simulink model "pidACC_bicycleModel"  (R2022a)
settings: Solver=FixedStepAuto  StartTime=0.0  StopTime=T  RelTol=1e-3
values from neighbouring files (symbols this model uses):
  o0_ego_1 = 0    [PreRun.m]
  o0_lead = 0    [PreRun.m]
  t_gap = 1.4    [PreRun.m]
  Ts = 1e-2    (= 0.01)    [PreRun.m]
  v0_ego_1 = 20/9    (= 2.22222222222)    [PreRun.m]
  v0_lead = 25/9    (= 2.77777777778)    [PreRun.m]
  x0_ego_1 = x0_lead - (10 + t_gap*v0_ego_1)    (= 56.8888888889)    [PreRun.m]
  x0_ego_2 = x0_ego_1 - (10 + t_gap*v0_ego_2)    (= 43.7777777778)    [PreRun.m]
  x0_lead = 70    [PreRun.m]
  y0_ego_1 = 0    [PreRun.m]
  y0_lead = 0    [PreRun.m]
undefined symbols (not defined in the file or in its folder): orient_kp
libraries: robotmobilelib x3
settings Model: Creator=The MathWorks, Inc.  LastModifiedBy=SAMEER TALWAR
settings SolverCC: AlgebraicLoopSolver=TrustRegion
settings DataIOCC: ReturnWorkspaceOutputs=off
settings DebuggingCC: UnconnectedInputMsg=warning  UnconnectedOutputMsg=warning  UnconnectedLineMsg=warning  SFMachineParentedDataDiag=warning  ArithmeticOperatorsInVariantConditions=warning
settings SFSimCC: SimUseLocalCustomCode=off  CustomCodeUndefinedFunction=UseInterfaceOnly
settings RTWCC: RTWUseLocalCustomCode=off
settings CodeAppCC: StateflowObjectComments=on

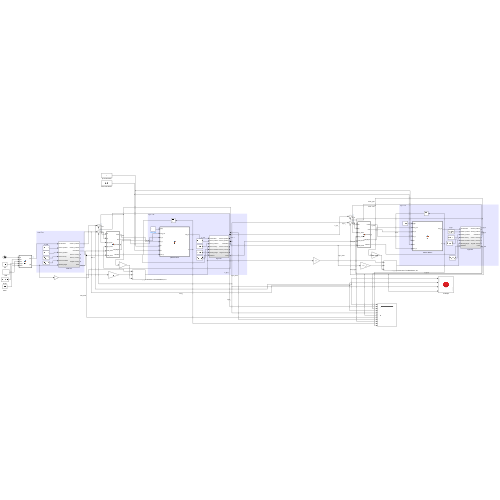
[thumbnail: Simulink's stored preview of the top-level diagram]
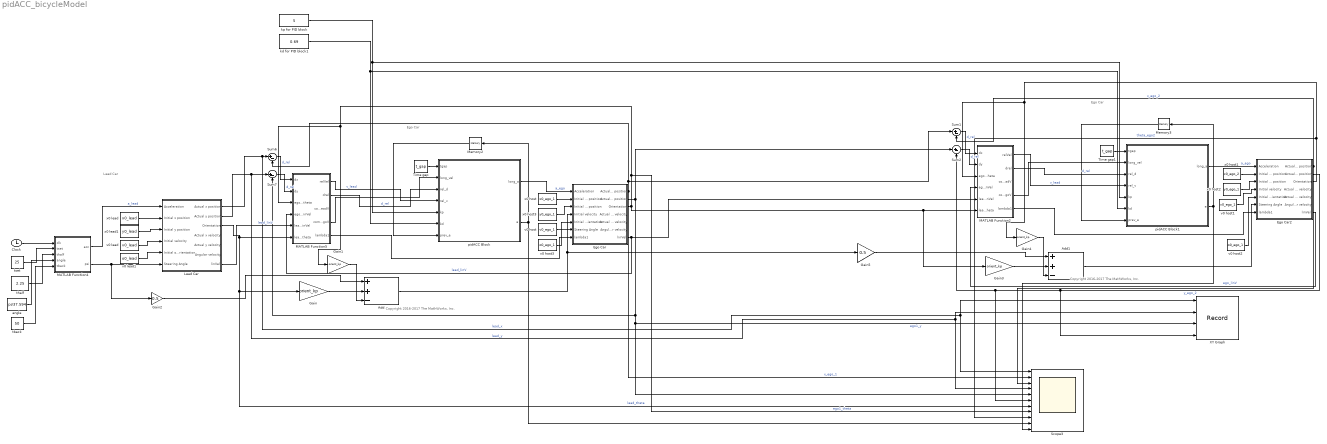
== system pidACC_bicycleModel ==
  note: Lead Car
  note: Ego Car
  note: Copyright 2016-2017 The MathWorks, Inc.
  note: Ego Car
  note: Copyright 2016-2017 The MathWorks, Inc.
  Add : Sum  Inputs=++-
  Add1 : Sum  Inputs=++-
  Clock : Clock
  Ego Car : Subsystem
  Ego Car2 : Subsystem
  Gain{,1,3..4} (4 alike) : Gain  Gain=orient_kp
  Gain2 : Gain  Gain=0.5
  Gain5 : Gain  Gain=0.5
  Lead Car : Subsystem
  MATLAB Function2 : MATLAB Function  TreatAsAtomicUnit=on
  MATLAB Function4 : MATLAB Function  TreatAsAtomicUnit=on
  MATLAB Function5 : MATLAB Function  TreatAsAtomicUnit=on
  Memory2 : Memory
  Memory3 : Memory
  Scope3 : Scope  NumInputPorts=11
  Sum{1..2,6..7} (4 alike) : Sum  Inputs=|+-
  Time gap : Constant  Value=t_gap  SampleTime=Ts
  Time gap1 : Constant  Value=t_gap  SampleTime=Ts
  XY Graph : Record  FileSettingsInternal="{\"entries\":[{\"content\":{\"excelSettings\":{\"content\":{},\"type\":\"Streamout.ExcelSettings\"}},\"type\":\"Streamout.FileSettingStorage\",\"uuid\":\"1b9ff1ee-6e9a-48d4-b5ec-83ee6443e3a1\"}],\"packageUris\":[\"http://schema.mathworks.com/mf0/streamout_blocks/R2020a\"],\"version\":\"1.0\"}"  Layout=[1 1]  SignalsInternal="{\"entries\":[{\"content\":{\"signals\":[{\"content\":{\"blockPath\":[\"pidACC_bicycleModel/XY Graph\"],\"channel\":[],\"dimensions\":[1],\"domain\":\"pidACC_bicycleModel/XY Graph\",\"lineColor\":\"#a2142f\",\"plots\":[1],\"port\":1,\"sid\":[\"\"],\"signalID\":5045,\"signalName\":\"lead_x\"},\"type\":\"RecordBlkView.Signal\",\"uuid\":\"68c1d946-6dfd-467f-94d7-86fec577fb75\"},{\"content\":{\"blockPath\":[\"pidACC_bicycleModel/XY Graph\"],\"channel\":[],\"dimensions\":[1],\"domain\":\"pidACC_bicycleModel/XY Graph\",\"lineColor\":\"#139fff\",\"plots\":[1],\"port\":2,\"sid\":[\"\"],\"signalID\":5049,\"signalName\":\"lead_y\"},\"type\":\"RecordBlkView.Signal\",\"uuid\":\"3b72477f-7d42-42a3-9da7-14649b2eb44c\"},{\"content\":{\"blockPath\":[\"pidACC_bicycleModel/XY Graph\"],\"channel\":[],\"dimensions\":[1],\"domain\":\"pidACC_bicycleModel/XY Graph\",\"lineColor\":\"#0072bd\",\"plots\":[1],\"port\":3,\"sid\":[\"\"],\"signalID\":5053,\"signalName\":\"ego1_y\"},\"type\":\"RecordBlkView.Signal\",\"uuid\":\"4297b810-ad1e-4c4e-9f18-f083e153cc8f\"},{\"content\":{\"blockPath\":[\"pidACC_bicycleModel/XY Graph\"],\"channel\":[],\"dimensions\":[1],\"domain\":\"pidACC_bicycleModel/XY Graph\",\"lineColor\":\"#d95319\",\"plots\":[1],\"port\":4,\"sid\":[\"\"],\"signalID\":5057,\"signalName\":\"y_ego_2\"},\"type\":\"RecordBlkView.Signal\",\"uuid\":\"56355f5a-31c0-4b9c-a448-66663cde7c29\"}]},\"type\":\"RecordBlkView.InputSignals\",\"uuid\":\"2dcac56b-3057-4ba9-be3c-f8c524bad982\"}],\"packageUris\":[\"http://schema.mathworks.com/mf0/streamout_blocks/R2020a\"],\"version\":\"1.0\"}"  VisualizationBindings="{\"xyplotplugin\":{\"info\":[{\"series\":[{\"bindingParametersList\":[{\"parameter\":\"X-Axis\",\"signalID\":5045,\"signalName\":\"lead_x\"},{\"parameter\":\"Y-Axis\",\"signalID\":5049,\"signalName\":\"lead_y\"}],\"seriesID\":62641},{\"bindingParametersList\":[{\"parameter\":\"X-Axis\",\"signalID\":5045,\"signalName\":\"lead_x\"},{\"parameter\":\"Y-Axis\",\"signalID\":5053,\"signalName\":\"ego1_y\"}],\"seriesID\":200},{\"bindingParametersList\":[{\"parameter\":\"X-Axis\",\"signalID\":5045,\"signalName\":\"lead_x\"},{\"parameter\":\"Y-Axis\",\"signalID\":5057,\"signalName\":\"y_ego_2\"}],\"seriesID\":276}],\"subplotID\":1}]}}"  CompatibilityTag=XY
  angle : Constant  Value=pi/37.594
  kd for PID block1 : Constant  Value=0.69
  kp for PID block : Constant  Value=5
  pidACC Block : MATLAB Function  TreatAsAtomicUnit=on
  pidACC Block1 : MATLAB Function  TreatAsAtomicUnit=on
  tback : Constant  Value=50
  thalf : Constant  Value=2.25
  tset : Constant  Value=25
  v0 host : Constant  Value=v0_ego_1  SampleTime=Ts
  v0 host1 : Constant  Value=v0_ego_1  SampleTime=Ts
  v0 host2 : Constant  Value=o0_ego_1  SampleTime=Ts
  v0 host3 : Constant  Value=o0_ego_1  SampleTime=Ts
  v0 lead : Constant  Value=v0_lead  SampleTime=Ts
  v0 lead1 : Constant  Value=o0_lead  SampleTime=Ts
  x0 host : Constant  Value=x0_ego_1  SampleTime=Ts
  x0 host1 : Constant  Value=x0_ego_2  SampleTime=Ts
  x0 host2 : Constant  Value=y0_ego_1  SampleTime=Ts
  x0 host3 : Constant  Value=y0_ego_1  SampleTime=Ts
  x0 lead : Constant  Value=x0_lead  SampleTime=Ts
  x0 lead1 : Constant  Value=y0_lead  SampleTime=Ts
  wires:
  x0 lead/1 -> Lead Car/2(Initial x position)
  v0 lead/1 -> Lead Car/4(Initial velocity)
  x0 host/1 -> Ego Car/2(Initial x position)
  pidACC Block/1(long_a) -> Ego Car/1(Acceleration)  "a_ego"
  MATLAB Function5/2(drel) -> pidACC Block/3(rel_d)  "d_rel"
  Time gap/1 -> pidACC Block/1(tgap)
  Ego Car/1(Actual x position) -> Sum1/1, Sum6/2, Scope3/2  "x_ego_1"
  MATLAB Function4/1(acc) -> Lead Car/1(Acceleration)  "a_lead"
  x0 host3/1 -> Ego Car/3(Initial y position)
  v0 host3/1 -> Ego Car/5(Initial orientation)
  Add/1 -> Gain5/1, Ego Car/6(Steering Angle)
  Clock/1 -> MATLAB Function4/1(clk)
  tset/1 -> MATLAB Function4/2(tset)
  thalf/1 -> MATLAB Function4/3(thalf)
  angle/1 -> MATLAB Function4/4(angle)
  MATLAB Function4/2(psi) -> Gain2/1, Lead Car/6(Steering Angle)
  x0 lead1/1 -> Lead Car/3(Initial y position)
  v0 lead1/1 -> Lead Car/5(Initial orientation)
  Lead Car/1(Actual x position) -> Scope3/1, XY Graph/1, Sum6/1  "lead_x"
  Lead Car/2(Actual y position) -> Scope3/4, XY Graph/2, Sum7/1  "lead_y"
  Sum6/1 -> MATLAB Function5/1(dx)  "d_rel"
  Sum7/1 -> MATLAB Function5/2(dy)  "d_rel"
  Lead Car/7(linVel) -> MATLAB Function5/5(lead_linVel)  "lead_linV"
  Lead Car/3(Orientation) -> Scope3/7, Gain/1, MATLAB Function5/6(lead_theta)  "lead_theta"
  MATLAB Function5/1(relVel) -> pidACC Block/4(rel_v)  "v_lead"
  MATLAB Function5/4(compEgoV) -> pidACC Block/2(long_vel)
  MATLAB Function5/5(lambda1) -> Ego Car/7(lambda1)
  Gain/1 -> Add/2
  Gain1/1 -> Add/3
  Gain2/1 -> Add/1
  Ego Car/7(linVel) -> MATLAB Function2/5(lead_linVel), MATLAB Function5/4(ego_linVel)  "lead_linV"
  Ego Car2/2(Actual y position) -> XY Graph/4, Sum2/2, Scope3/6  "y_ego_2"
  MATLAB Function2/5(lambda1) -> Ego Car2/7(lambda1)
  Gain3/1 -> Add1/2
  Gain4/1 -> Add1/3
  x0 host1/1 -> Ego Car2/2(Initial x position)
  Sum1/1 -> MATLAB Function2/1(dx)  "d_rel"
  Sum2/1 -> MATLAB Function2/2(dy)  "d_rel"
  Ego Car2/3(Orientation) -> Scope3/9, Gain4/1, MATLAB Function2/3(ego_theta)  "theta_ego2"
  Ego Car/3(Orientation) -> Gain3/1, MATLAB Function2/6(lead_theta), Scope3/8, Gain1/1, MATLAB Function5/3(ego_theta)  "ego1_theta"
  v0 host2/1 -> Ego Car2/5(Initial orientation)
  x0 host2/1 -> Ego Car2/3(Initial y position)
  v0 host/1 -> Ego Car/4(Initial velocity)
  Ego Car/2(Actual y position) -> Sum2/1, Scope3/5, XY Graph/3, Sum7/2  "ego1_y"
  MATLAB Function2/4(compEgoV) -> pidACC Block1/2(long_vel)
  MATLAB Function2/1(relVel) -> pidACC Block1/4(rel_v)  "v_lead"
  Add1/1 -> Ego Car2/6(Steering Angle)
  Ego Car2/7(linVel) -> MATLAB Function2/4(ego_linVel)  "ego_linV"
  v0 host1/1 -> Ego Car2/4(Initial velocity)
  MATLAB Function2/2(drel) -> pidACC Block1/3(rel_d)  "d_rel"
  pidACC Block1/1(long_a) -> Ego Car2/1(Acceleration)  "a_ego"
  Ego Car2/1(Actual x position) -> Scope3/3, Sum1/2  "x_ego_2"
  Time gap1/1 -> pidACC Block1/1(tgap)
  Gain5/1 -> Add1/1
  tback/1 -> MATLAB Function4/5(tback)
  pidACC Block/2(e) -> Memory2/1, Scope3/10
  Memory2/1 -> pidACC Block/7(prev_e)
  kd for PID block1/1 -> pidACC Block1/6(kd), pidACC Block/6(kd)
  kp for PID block/1 -> pidACC Block1/5(kp), pidACC Block/5(kp)
  pidACC Block1/2(e) -> Scope3/11, Memory3/1
  Memory3/1 -> pidACC Block1/7(prev_e)

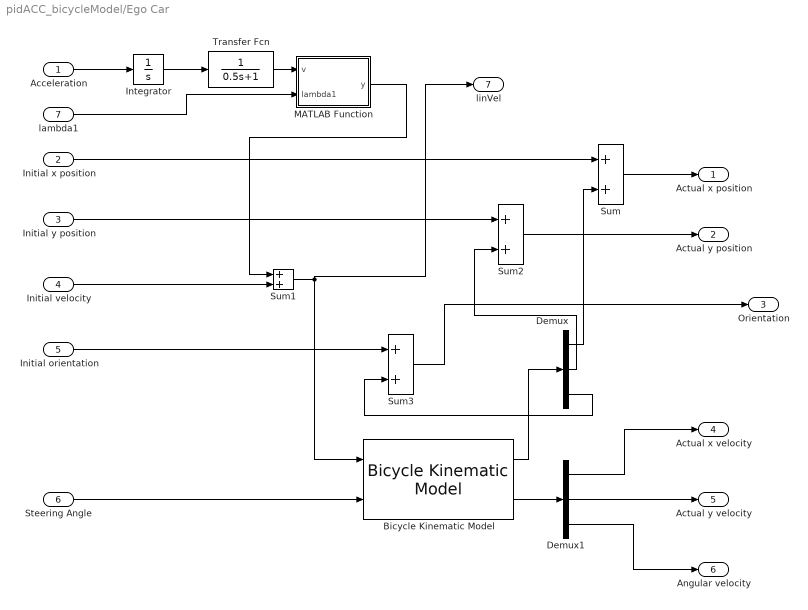
== system pidACC_bicycleModel/Ego Car ==
  Acceleration : Inport
  Initial x position : Inport  Port=2
  Initial y position : Inport  Port=3
  Initial velocity : Inport  Port=4
  Initial orientation : Inport  Port=5
  Steering Angle : Inport  Port=6
  lambda1 : Inport  Port=7
  Bicycle Kinematic Model : robotmobilelib/Bicycle Kinematic Model  VehicleInputs=Vehicle Speed & Steering Angle  WheelBase=1  VehicleSpeedRange=[-inf inf]  MaxSteeringAngle=pi/4  InitialState=[0; 0; 0]  SimulateUsing=Interpreted execution
      settings: SourceProductBaseCode=RO
  Demux : Demux  Outputs=3
  Demux1 : Demux  Outputs=3
  Integrator : Integrator
  MATLAB Function : MATLAB Function  TreatAsAtomicUnit=on
  Sum{,1..3} (4 alike) : Sum
  Transfer Fcn : TransferFcn  Denominator=[0.5 1]
  Actual x position : Outport  VectorParamsAs1DForOutWhenUnconnected=off
  Actual y position : Outport  Port=2
  Orientation : Outport  Port=3
  Actual x velocity : Outport  Port=4  VectorParamsAs1DForOutWhenUnconnected=off
  Actual y velocity : Outport  Port=5
  Angular velocity : Outport  Port=6
  linVel : Outport  Port=7
  wires:
  Initial velocity/1 -> Sum1/2
  Sum/1 -> Actual x position/1
  Integrator/1 -> Transfer Fcn/1
  Acceleration/1 -> Integrator/1
  Initial x position/1 -> Sum/1
  Demux/1 -> Sum/2
  Bicycle Kinematic Model/1 -> Demux/1
  Sum1/1 -> linVel/1, Bicycle Kinematic Model/1
  Steering Angle/1 -> Bicycle Kinematic Model/2
  Bicycle Kinematic Model/2 -> Demux1/1
  Demux1/1 -> Actual x velocity/1
  Demux1/2 -> Actual y velocity/1
  Demux1/3 -> Angular velocity/1
  Initial y position/1 -> Sum2/1
  Demux/2 -> Sum2/2
  Sum2/1 -> Actual y position/1
  Initial orientation/1 -> Sum3/1
  Demux/3 -> Sum3/2
  Sum3/1 -> Orientation/1
  Transfer Fcn/1 -> MATLAB Function/1(v)
  lambda1/1 -> MATLAB Function/2(lambda1)
  MATLAB Function/1(y) -> Sum1/1

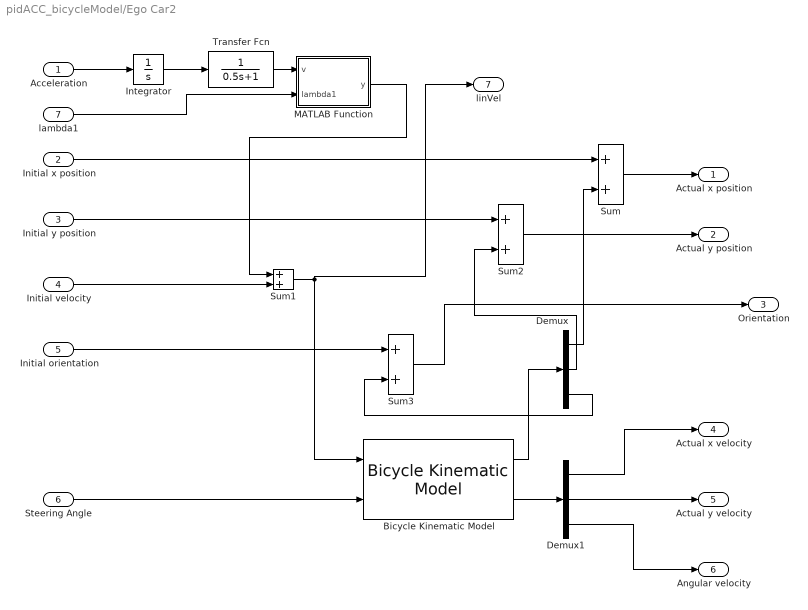
== system pidACC_bicycleModel/Ego Car2 ==
  Acceleration : Inport
  Initial x position : Inport  Port=2
  Initial y position : Inport  Port=3
  Initial velocity : Inport  Port=4
  Initial orientation : Inport  Port=5
  Steering Angle : Inport  Port=6
  lambda1 : Inport  Port=7
  Bicycle Kinematic Model : robotmobilelib/Bicycle Kinematic Model  VehicleInputs=Vehicle Speed & Steering Angle  WheelBase=1  VehicleSpeedRange=[-inf inf]  MaxSteeringAngle=pi/4  InitialState=[0; 0; 0]  SimulateUsing=Interpreted execution
      settings: SourceProductBaseCode=RO
  Demux : Demux  Outputs=3
  Demux1 : Demux  Outputs=3
  Integrator : Integrator
  MATLAB Function : MATLAB Function  TreatAsAtomicUnit=on
  Sum{,1..3} (4 alike) : Sum
  Transfer Fcn : TransferFcn  Denominator=[0.5 1]
  Actual x position : Outport  VectorParamsAs1DForOutWhenUnconnected=off
  Actual y position : Outport  Port=2
  Orientation : Outport  Port=3
  Actual x velocity : Outport  Port=4  VectorParamsAs1DForOutWhenUnconnected=off
  Actual y velocity : Outport  Port=5
  Angular velocity : Outport  Port=6
  linVel : Outport  Port=7
  wires:
  Initial velocity/1 -> Sum1/2
  Sum/1 -> Actual x position/1
  Integrator/1 -> Transfer Fcn/1
  Acceleration/1 -> Integrator/1
  Initial x position/1 -> Sum/1
  Demux/1 -> Sum/2
  Bicycle Kinematic Model/1 -> Demux/1
  Sum1/1 -> linVel/1, Bicycle Kinematic Model/1
  Steering Angle/1 -> Bicycle Kinematic Model/2
  Bicycle Kinematic Model/2 -> Demux1/1
  Demux1/1 -> Actual x velocity/1
  Demux1/2 -> Actual y velocity/1
  Demux1/3 -> Angular velocity/1
  Initial y position/1 -> Sum2/1
  Demux/2 -> Sum2/2
  Sum2/1 -> Actual y position/1
  Initial orientation/1 -> Sum3/1
  Demux/3 -> Sum3/2
  Sum3/1 -> Orientation/1
  Transfer Fcn/1 -> MATLAB Function/1(v)
  lambda1/1 -> MATLAB Function/2(lambda1)
  MATLAB Function/1(y) -> Sum1/1

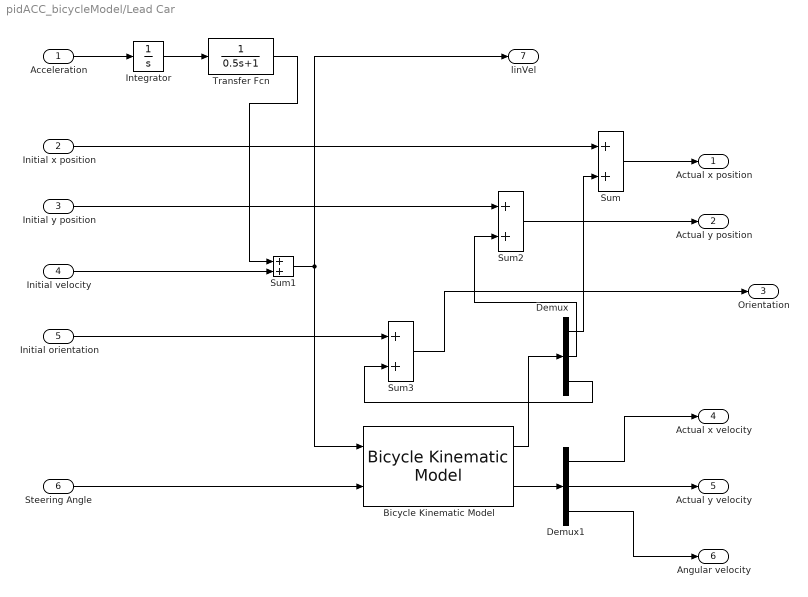
== system pidACC_bicycleModel/Lead Car ==
  Acceleration : Inport
  Initial x position : Inport  Port=2
  Initial y position : Inport  Port=3
  Initial velocity : Inport  Port=4
  Initial orientation : Inport  Port=5
  Steering Angle : Inport  Port=6
  Bicycle Kinematic Model : robotmobilelib/Bicycle Kinematic Model  VehicleInputs=Vehicle Speed & Steering Angle  WheelBase=1  VehicleSpeedRange=[-inf inf]  MaxSteeringAngle=pi/4  InitialState=[0; 0; 0]  SimulateUsing=Interpreted execution
      settings: SourceProductBaseCode=RO
  Demux : Demux  Outputs=3
  Demux1 : Demux  Outputs=3
  Integrator : Integrator
  Sum{,1..3} (4 alike) : Sum
  Transfer Fcn : TransferFcn  Denominator=[0.5 1]
  Actual x position : Outport  VectorParamsAs1DForOutWhenUnconnected=off
  Actual y position : Outport  Port=2
  Orientation : Outport  Port=3
  Actual x velocity : Outport  Port=4  VectorParamsAs1DForOutWhenUnconnected=off
  Actual y velocity : Outport  Port=5
  Angular velocity : Outport  Port=6
  linVel : Outport  Port=7
  wires:
  Bicycle Kinematic Model/1 -> Demux/1
  Sum3/1 -> Orientation/1
  Steering Angle/1 -> Bicycle Kinematic Model/2
  Demux1/1 -> Actual x velocity/1
  Demux/1 -> Sum/2
  Demux/3 -> Sum3/2
  Demux1/2 -> Actual y velocity/1
  Initial orientation/1 -> Sum3/1
  Demux/2 -> Sum2/2
  Sum2/1 -> Actual y position/1
  Demux1/3 -> Angular velocity/1
  Bicycle Kinematic Model/2 -> Demux1/1
  Sum1/1 -> linVel/1, Bicycle Kinematic Model/1
  Integrator/1 -> Transfer Fcn/1
  Acceleration/1 -> Integrator/1
  Transfer Fcn/1 -> Sum1/1
  Initial y position/1 -> Sum2/1
  Sum/1 -> Actual x position/1
  Initial x position/1 -> Sum/1
  Initial velocity/1 -> Sum1/2

== matlab function pidACC_bicycleModel/Ego Car/MATLAB Function ==
  data: y output; v input; lambda1 input
function y = fcn(v, lambda1)

y = v*sec(lambda1);

== matlab function pidACC_bicycleModel/pidACC Block1 ==
  data: tgap input; long_a output; long_vel input; rel_d input; rel_v input; e output; kp input; kd input; prev_e input
function [long_a,e] = fcn(tgap, long_vel, rel_d, rel_v, kp, kd, prev_e)
dt=0.01;
dsafe = 10 + (tgap*long_vel);
e = rel_d - dsafe;
long_a = kp*e + kd*(e-prev_e)/dt;

== matlab function pidACC_bicycleModel/Ego Car2/MATLAB Function ==
  data: y output; v input; lambda1 input
function y = fcn(v, lambda1)

y = v*sec(lambda1);

== matlab function pidACC_bicycleModel/MATLAB Function4 ==
  data: clk input; acc output; tset input; thalf input; angle input; psi output; tback input
function [acc,psi] = fcn(clk,tset,thalf, angle, tback)
if clk>tset && clk<(tset+thalf)
    psi = angle;
elseif clk>(tset+thalf) && clk<(tset + 2*thalf)
    psi = -angle;
elseif clk>(tset + 2*thalf) && clk<(tback)
    psi = 0;
elseif clk>(tback) && clk<(tback+thalf)
    psi = -angle;
elseif clk>(tback+thalf) && clk<(tback+ 2*thalf)
    psi = angle;
else psi=0;
end
acc=0;

== matlab function pidACC_bicycleModel/MATLAB Function5 ==
  data: relVel output; dx input; drel output; dy input; ego_theta input; ego_linVel input; lead_linVel input; lead_theta input; compLeadV output; compEgoV output; lambda1 output
function [relVel,drel,compLeadV, compEgoV, lambda1] = fcn(dx,dy, ego_theta, ego_linVel,lead_linVel, lead_theta)
drel = sqrt(dx^2 + dy^2);
lambda1 = atan(dy/dx) - ego_theta;
lambda2 = atan(dy/dx) - lead_theta;
relVel = lead_linVel*cos(lambda2) - ego_linVel*cos(lambda1);
compLeadV = lead_linVel*cos(lambda2);
compEgoV = ego_linVel*cos(lambda1);

== matlab function pidACC_bicycleModel/MATLAB Function2 ==
  data: relVel output; dx input; drel output; dy input; ego_theta input; ego_linVel input; lead_linVel input; lead_theta input; compLeadV output; compEgoV output; lambda1 output
function [relVel,drel,compLeadV, compEgoV, lambda1] = fcn(dx,dy, ego_theta, ego_linVel,lead_linVel, lead_theta)
drel = sqrt(dx^2 + dy^2);
lambda1 = atan(dy/dx) - ego_theta;
lambda2 = atan(dy/dx) - lead_theta;
relVel = lead_linVel*cos(lambda2) - ego_linVel*cos(lambda1);
compLeadV = lead_linVel*cos(lambda2);
compEgoV = ego_linVel*cos(lambda1);

== matlab function pidACC_bicycleModel/pidACC Block ==
  data: tgap input; long_a output; long_vel input; rel_d input; rel_v input; e output; kp input; kd input; prev_e input
function [long_a,e] = fcn(tgap, long_vel, rel_d, rel_v, kp, kd, prev_e)
dt=0.01;
dsafe = 10 + (tgap*long_vel);
e = rel_d - dsafe;
long_a = kp*e + kd*(e-prev_e)/dt;
